simulink model "oneDOF_PDcontrol"  (R2022a)
settings: Solver=VariableStepAuto  StartTime=0.0  StopTime=10  RelTol=1e-3
model workspace (MAT data in the model file):
  D = 1
  K = 4
  m = 2
  v0 = 0
  x0 = [10 0]
  x_des = [5 0]
settings Model: Creator=Tommaso  LastModifiedBy=Tommaso

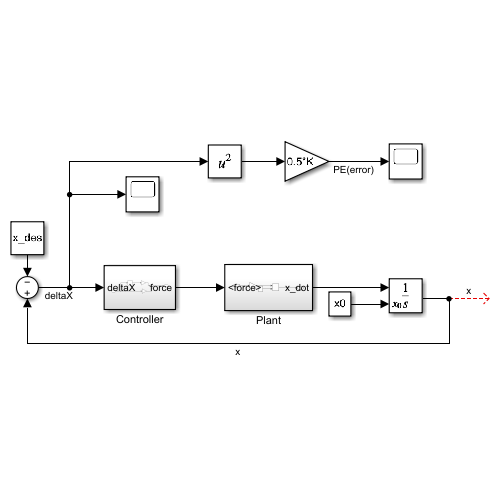
[thumbnail: Simulink's stored preview of the top-level diagram]
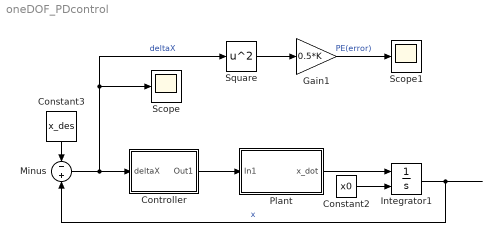
== system oneDOF_PDcontrol ==
  Constant2 : Constant  Value=x0
  Constant3 : Constant  Value=x_des
  Controller : Subsystem
  Gain1 : Gain  Gain=0.5*K
  Integrator1 : Integrator  InitialConditionSource=external
  Minus : Sum  Inputs=-+
  Plant : Subsystem
  Scope : Scope
  Scope1 : Scope
  Square : Math  Operator=square
  wires:
  Square/1 -> Gain1/1
  Constant3/1 -> Minus/1
  Gain1/1 -> Scope1/1  "PE(error)"
  Minus/1 -> Controller/1(deltaX), Square/1, Scope/1  "deltaX"
  Integrator1/1 -> Minus/2  "x"
  Constant2/1 -> Integrator1/2
  Controller/1(Out1) -> Plant/1(In1)
  Plant/1(x_dot) -> Integrator1/1

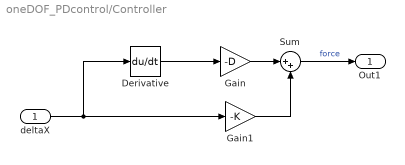
== system oneDOF_PDcontrol/Controller ==
  deltaX : Inport
  Derivative : Derivative
  Gain : Gain  Gain=-D
  Gain1 : Gain  Gain=-K
  Sum : Sum  Inputs=|++
  Out1 : Outport
  wires:
  deltaX/1 -> Derivative/1, Gain1/1
  Gain/1 -> Sum/1
  Gain1/1 -> Sum/2
  Sum/1 -> Out1/1  "force"
  Derivative/1 -> Gain/1

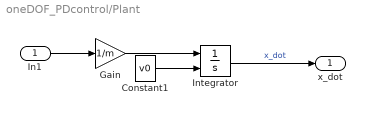
== system oneDOF_PDcontrol/Plant ==
  In1 : Inport
  Constant1 : Constant  Value=v0
  Gain : Gain  Gain=1/m
  Integrator : Integrator  InitialConditionSource=external
  x_dot : Outport
  wires:
  Gain/1 -> Integrator/1
  Constant1/1 -> Integrator/2
  Integrator/1 -> x_dot/1  "x_dot"
  In1/1 -> Gain/1
